simulink model "ControlSys_v17_Demo"  (R2020b)
settings: Solver=VariableStepAuto  StartTime=0  StopTime=SimTime  FixedStep=0.01  MaxStep=0.01  RelTol=1e-4
undefined symbols (not defined in the file): CDTRR, CST, initTemp_deg, Nm1, ODTRR, SST, Tout, Tset, Tss
libraries: simulink x3, slident x1, pid_lib x1
settings Model: OrderedModelArguments=off  Creator=Arwa Abougharib  LastModifiedBy=Arwa Abougharib
settings SolverCC: AlgebraicLoopSolver=LineSearch  AutoInsertRateTranBlk=on  InsertRTBMode=Never (minimum delay)
settings DataIOCC: LimitDataPoints=on  SaveFormat=StructureWithTime  SaveOutput=off  SaveTime=off
settings OptimizationCC: ExpressionDepthLimit=2147483647  LifeSpan=1
settings DebuggingCC: MergeDetectMultiDrivingBlocksExec=none  FcnCallInpInsideContextMsg=warning  AllowSymbolicDim=off  StateNameClashWarn=warning  SFUnexpectedBacktrackingDiag=warning  SFNoUnconditionalDefaultTransitionDiag=warning  SFExecutionAtInitializationDiag=none  ArithmeticOperatorsInVariantConditions=warning
settings SFSimCC: SimUseLocalCustomCode=off  CustomCodeUndefinedFunction=UseInterfaceOnly
settings RTWCC: RTWUseLocalCustomCode=off
settings CodeAppCC: StateflowObjectComments=on
settings GRTTargetCC: TargetLangStandard=C89/C90 (ANSI)  CombineOutputUpdateFcns=off  GRTInterface=on

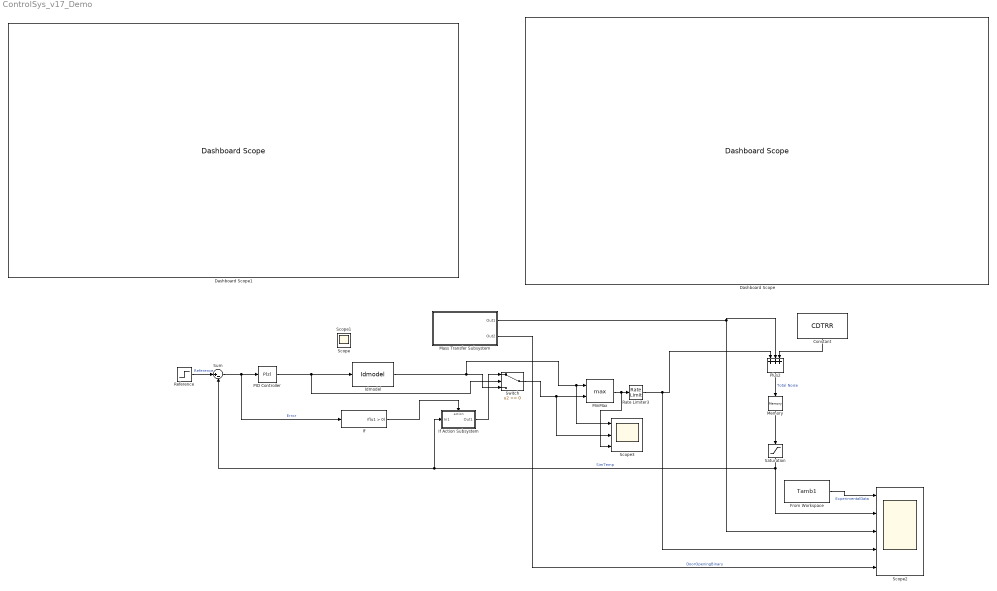
== system ControlSys_v17_Demo ==
  Constant : Constant  Value=CDTRR  SampleTime=1
  Dashboard Scope : DashboardScope
  Dashboard Scope1 : DashboardScope
  From Workspace : FromWorkspace  VariableName=Tamb1  SampleTime=SST  Interpolate=off  OutputAfterFinalValue=Cyclic repetition
  Idmodel : slident/Models/Idmodel  sys=sys  IC=sys.Report.Parameters.X0  noi=off  seed=[]
      settings: SourceProductBaseCode=ID
  If : If  ShowElse=off
  If Action Subsystem : Subsystem  TreatAsAtomicUnit=on
  Mass Transfer Subsystem : Subsystem
  Memory : Memory  InitialCondition=initTemp_deg  InheritSampleTime=on
  MinMax : MinMax  Function=max  Inputs=2
  PID Controller : pid_lib/PID Controller  Controller=P  Form=Parallel  TimeDomain=Discrete-time  UseExternalTs=off  SampleTime=CST  IntegratorMethod=Forward Euler  FilterMethod=Forward Euler  ControllerParametersSource=internal  P=1  I=0  D=0  UseFilter=on  N=0.0507941980313757  TunerSelectOption=Transfer Function Based (PID Tuner App)  InitialConditionSource=internal  InitialConditionForIntegrator=0  InitialConditionForFilter=0  DifferentiatorICPrevScaledInput=0  ExternalReset=none  TrackingMode=off  Kt=2  LimitOutput=on  SatLimitsSource=internal  UpperSaturationLimit=0  LowerSaturationLimit=-inf  LinearizeAsGain=off  AntiWindupMode=none  Kb=1  RndMeth=Nearest  POutMin=[]  POutMax=[]  IOutMin=[]  IOutMax=[]  DOutMin=[]  DOutMax=[]  NOutMin=[]  NOutMax=[]  SumOutMin=[]  SumOutMax=[]  SaturationOutMin=[]  SaturationOutMax=[]  PParamMin=[]  PParamMax=[]  IParamMin=[]  IParamMax=[]  DParamMin=[]  DParamMax=[]  NParamMin=[]  NParamMax=[]  KbParamMin=[]  KbParamMax=[]  KtParamMin=[]  KtParamMax=[]  KbOutMin=[]  KbOutMax=[]  KtOutMin=[]  KtOutMax=[]  IntegratorOutMin=[]  IntegratorOutMax=[]  FilterOutMin=[]  FilterOutMax=[]  SumI1OutMin=[]  SumI1OutMax=[]  SumI2OutMin=[]  SumI2OutMax=[]  SumI3OutMin=[]  SumI3OutMax=[]  SumI4OutMin=[]  SumI4OutMax=[]  SumDOutMin=[]  SumDOutMax=[]  DifferentiatorOutMin=[]  DifferentiatorOutMax=[]  FilterDiffOutCoefMin=[]  FilterDiffOutCoefMax=[]  ReciprocalOutMin=[]  ReciprocalOutMax=[]  SumDenOutMin=[]  SumDenOutMax=[]  SumNumOutMin=[]  SumNumOutMax=[]  DivideOutMin=[]  DivideOutMax=[]  UdiffTsProdOutMin=[]  UdiffTsProdOutMax=[]  NTsProdOutMin=[]  NTsProdOutMax=[]  UintegralTsProdOutMin=[]  UintegralTsProdOutMax=[]  UngainTsProdOutMin=[]  UngainTsProdOutMax=[]  IntegratorContinuousStateAttributes=''  IntegratorStateMustResolveToSignalObject=off  IntegratorRTWStateStorageClass=Auto  FilterContinuousStateAttributes=''  FilterStateMustResolveToSignalObject=off  FilterRTWStateStorageClass=Auto  ParallelPVariant=InternalParameters  IdealPVariant=Disabled  IVariant=Disabled  DVariant=Disabled  IntegratorVariant=Disabled  SatVariant=Enabled  AWVariant=Disabled  PCopyVariant=Disabled  TRVariant=Disabled  FdbkBlocksVariant=Forward  IdealPFdbkVariant=Disabled  SatFdbkVariant=Disabled  DerivativeFilterVariant=Disabled  NVariant=Disabled  NCopyVariant=Disabled_SignalSpec  FilterICVariant=Disabled  IntegratorICVariant=Disabled  ExternalResetVariant=Disabled  TRSumVariant=Passthrough  SumFdbkVariant=Disabled  SumVariant=Passthrough_P  TsampFilterVariant=InternalTs  TsampNgainVariant=Passthrough  TsampIntegralVariant=Disabled_SignalSpec  ExternalSaturationOutDataTypeStr=Inherit: Same as second input
  Plus2 : Sum  Inputs=+++
  Rate Limiter3 : RateLimiter  RisingSlewLimit=CDTRR  FallingSlewLimit=-CDTRR
  Reference : Step  Time=0  Before=Tset  After=Tset  SampleTime=0
  Saturation : Saturate  UpperLimit=Tout  LowerLimit=-inf
  Scope2 : Scope  NumInputPorts=5
  Scope3 : Scope  NumInputPorts=3
  Sum : Sum  Inputs=|+-
  Switch : Switch
  Scope : Scope
  Scope1 : Scope
  wires:
  Reference/1 -> Sum/1  "Reference"
  Plus2/1 -> Memory/1  "Total Noise"
  Constant/1 -> Plus2/3
  From Workspace/1 -> Scope2/1  "ExperimentalData"
  Sum/1 -> PID Controller/1, If/1  "Error"
  Saturation/1 -> If Action Subsystem/1(In1), Sum/2, Scope2/2  "SimTemp"
  If/1 -> If Action Subsystem/Action
  Memory/1 -> Saturation/1
  Mass Transfer Subsystem/1(Out1) -> Scope2/3, Plus2/2
  PID Controller/1 -> Switch/2, Idmodel/1
  Rate Limiter3/1 -> Scope2/4, Plus2/1
  Idmodel/1 -> Scope3/1, MinMax/1, Switch/3
  If Action Subsystem/1(Out1) -> Switch/1
  Mass Transfer Subsystem/2(Out2) -> Scope2/5  "DoorOpeningBinary"
  Switch/1 -> Scope3/2, MinMax/2
  MinMax/1 -> Scope3/3, Rate Limiter3/1

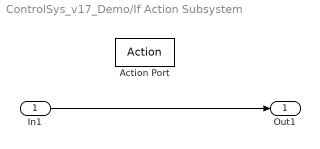
== system ControlSys_v17_Demo/If Action Subsystem ==
  In1 : Inport
  Action Port : ActionPort  ActionPortLabel=if(u1 > 0)
  Out1 : Outport
  wires:
  In1/1 -> Out1/1

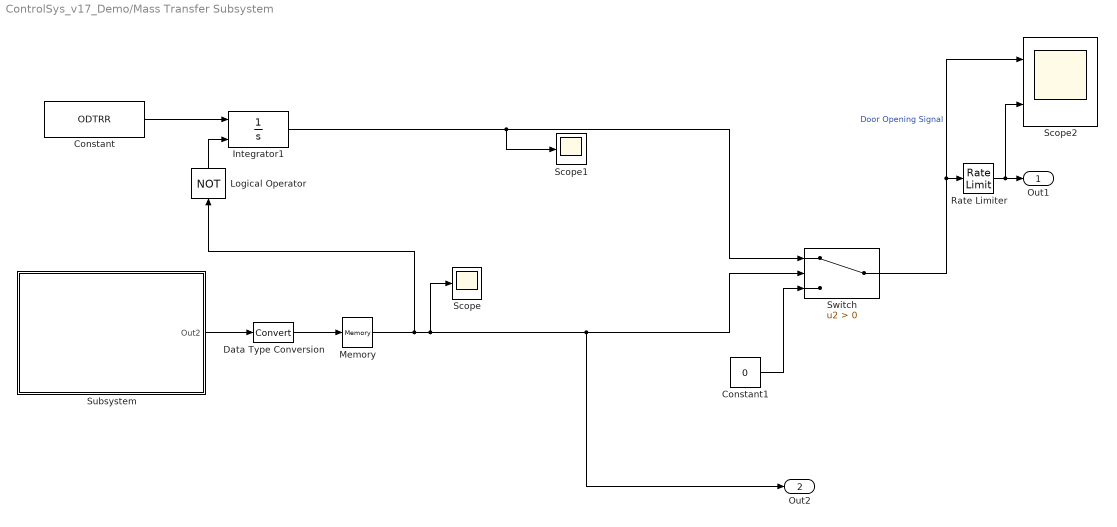
== system ControlSys_v17_Demo/Mass Transfer Subsystem ==
  Constant : Constant  Value=ODTRR  SampleTime=1
  Constant1 : Constant  Value=0
  Data Type Conversion : DataTypeConversion
  Integrator1 : Integrator  ExternalReset=level  LimitOutput=on  UpperSaturationLimit=Tout  LowerSaturationLimit=0  WrappedStateUpperValue=5  WrappedStateLowerValue=0
  Logical Operator : Logic  Operator=NOT  AllPortsSameDT=off  OutDataTypeStr=boolean
  Memory : Memory  InheritSampleTime=on
  Rate Limiter : RateLimiter  RisingSlewLimit=inf  FallingSlewLimit=-CDTRR  SampleTimeMode=inherited
  Scope : Scope
  Scope1 : Scope
  Scope2 : Scope  NumInputPorts=2
  Subsystem : Subsystem
  Switch : Switch  Criteria=u2 > Threshold
  Out1 : Outport
  Out2 : Outport  Port=2
  wires:
  Switch/1 -> Scope2/1, Rate Limiter/1  "Door Opening Signal"
  Subsystem/1(Out2) -> Data Type Conversion/1
  Data Type Conversion/1 -> Memory/1
  Constant/1 -> Integrator1/1
  Logical Operator/1 -> Integrator1/2
  Constant1/1 -> Switch/3
  Integrator1/1 -> Scope1/1, Switch/1
  Rate Limiter/1 -> Scope2/2, Out1/1
  Memory/1 -> Logical Operator/1, Scope/1, Out2/1, Switch/2

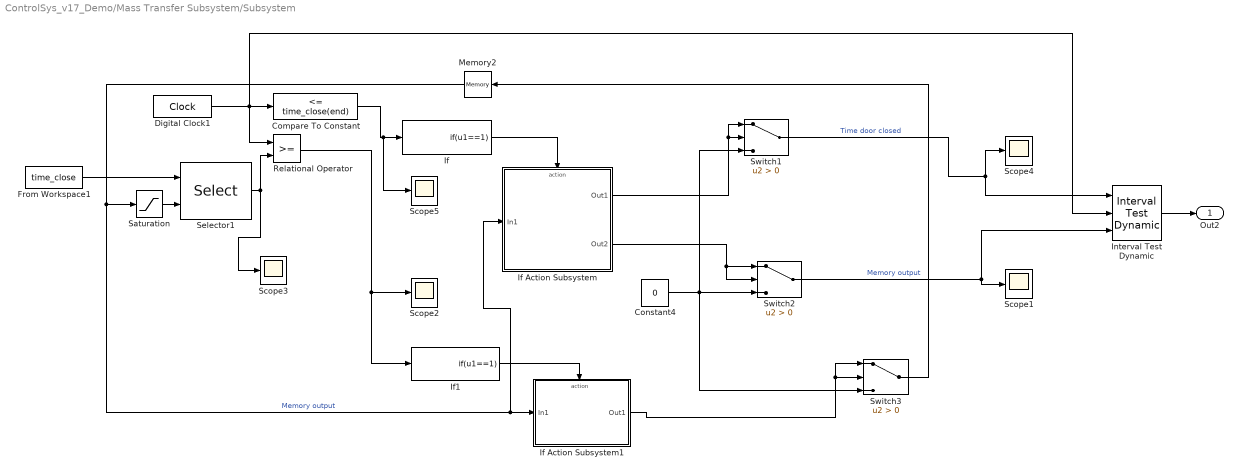
== system ControlSys_v17_Demo/Mass Transfer Subsystem/Subsystem ==
  Compare To Constant : simulink/Logic and Bit Operations/Compare To Constant  relop=<=  const=time_close(end)  OutDataTypeStr=boolean
  Constant4 : Constant  Value=0
  Digital Clock1 : DigitalClock  SampleTime=Tss
  From Workspace1 : FromWorkspace  VariableName=time_close  SampleTime=Tss  ZeroCross=off  OutputAfterFinalValue=Holding final value
  If : If  IfExpression=u1==1  ShowElse=off  ZeroCross=off
  If Action Subsystem : Subsystem  TreatAsAtomicUnit=on
  If Action Subsystem1 : Subsystem  TreatAsAtomicUnit=on
  If1 : If  IfExpression=u1==1  ShowElse=off  ZeroCross=off
  Interval Test Dynamic : simulink/Logic and Bit Operations/Interval Test Dynamic  IntervalClosedRight=on  IntervalClosedLeft=on  OutDataTypeStr=boolean
      settings: SourceProductBaseCode=SL
  Memory2 : Memory  InheritSampleTime=on  LinearizeAsDelay=on
  Relational Operator : RelationalOperator  OutDataTypeStr=boolean  RndMeth=Simplest
  Saturation : Saturate  UpperLimit=Nm1-1  LowerLimit=0
  Scope{1..5} (5 alike) : Scope
  Selector1 : Selector  IndexMode=Zero-based  InputPortWidth=Nm1  IndexOptions=Index vector (port)  Indices=[1 3]  OutputSizes=1
  Switch1 : Switch  Criteria=u2 > Threshold  RndMeth=Round
  Switch2 : Switch  Criteria=u2 > Threshold  RndMeth=Ceiling
  Switch3 : Switch  Criteria=u2 > Threshold
  Out2 : Outport
  wires:
  Constant4/1 -> Switch1/3, Switch3/3, Switch2/3
  Switch2/1 -> Interval Test Dynamic/3, Scope1/1  "Memory output"
  Switch1/1 -> Scope4/1, Interval Test Dynamic/1  "Time door closed"
  If Action Subsystem/2(Out2) -> Switch2/2, Switch2/1
  If Action Subsystem/1(Out1) -> Switch1/1, Switch1/2
  If Action Subsystem1/1(Out1) -> Switch3/1, Switch3/2
  Digital Clock1/1 -> Compare To Constant/1, Relational Operator/1, Interval Test Dynamic/2
  Interval Test Dynamic/1 -> Out2/1
  If/1 -> If Action Subsystem/Action
  From Workspace1/1 -> Selector1/1
  Switch3/1 -> Memory2/1
  Selector1/1 -> Relational Operator/2, Scope3/1
  Memory2/1 -> If Action Subsystem/1(In1), If Action Subsystem1/1(In1), Saturation/1  "Memory output"
  Saturation/1 -> Selector1/2
  If1/1 -> If Action Subsystem1/Action
  Compare To Constant/1 -> Scope5/1, If/1
  Relational Operator/1 -> Scope2/1, If1/1

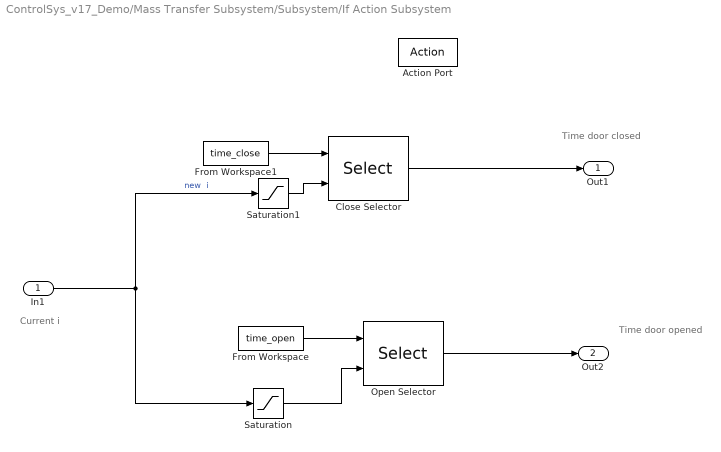
== system ControlSys_v17_Demo/Mass Transfer Subsystem/Subsystem/If Action Subsystem ==
  note: Current i
  note: Time door opened
  note: Time door closed
  In1 : Inport
  Action Port : ActionPort  ActionPortLabel=if(u1==1)
  Close Selector : Selector  IndexMode=Zero-based  InputPortWidth=Nm1  IndexOptions=Index vector (port)  Indices=[1 3]  OutputSizes=1
  From Workspace : FromWorkspace  VariableName=time_open  SampleTime=Tss  Interpolate=off  OutputAfterFinalValue=Holding final value
  From Workspace1 : FromWorkspace  VariableName=time_close  SampleTime=Tss  ZeroCross=off  OutputAfterFinalValue=Holding final value
  Open Selector : Selector  IndexMode=Zero-based  InputPortWidth=Nm1  IndexOptions=Index vector (port)  Indices=[1 3]  OutputSizes=1
  Saturation : Saturate  UpperLimit=Nm1-1  LowerLimit=-1  LinearizeAsGain=off
  Saturation1 : Saturate  UpperLimit=Nm1-1  LowerLimit=0  LinearizeAsGain=off
  Out1 : Outport
  Out2 : Outport  Port=2
  wires:
  Close Selector/1 -> Out1/1
  From Workspace/1 -> Open Selector/1
  Open Selector/1 -> Out2/1
  From Workspace1/1 -> Close Selector/1
  In1/1 -> Saturation1/1, Saturation/1  "new  i"
  Saturation/1 -> Open Selector/2
  Saturation1/1 -> Close Selector/2

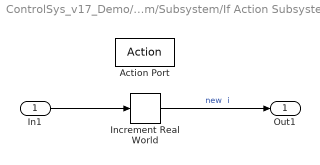
== system ControlSys_v17_Demo/Mass Transfer Subsystem/Subsystem/If Action Subsystem1 ==
  In1 : Inport
  Action Port : ActionPort  ActionPortLabel=if(u1==1)
  Increment Real World : simulink/Additional Math & Discrete/Additional Math: Increment - Decrement/Increment Real World
      settings: SourceProductBaseCode=SL
  Out1 : Outport
  wires:
  In1/1 -> Increment Real World/1
  Increment Real World/1 -> Out1/1  "new  i"
